simulink model "graph"  (R2015b)
settings: Solver=ode4  StartTime=0.0  StopTime=0.2  FixedStep=0.00002  RelTol=1e-3
settings Model: ExtModeTrigDuration=10000  Creator=husseinz  LastModifiedBy=husseinz
settings SolverCC: PositivePriorityOrder=on
settings RTWCC: SystemTargetFile=quarc_win64.tlc  TemplateMakefile=quarc_default_tmf  Description=QUARC Win64 Target
settings STFCustomTargetCC: TargetPreCompLibLocation=C:\ProgramData\QUARC\lib\2015b\win64\release  GeneratePreprocessorConditionals=Use local settings  CPPClassGenCompliant=off
settings GRTTargetCC: TargetPreCompLibLocation=C:\ProgramData\QUARC\lib\2015b\win64\release  ParMdlRefBuildCompliant=off  CompOptLevelCompliant=off  CombineOutputUpdateFcns=off  MatFileLogging=off  CPPClassGenCompliant=off  GRTInterface=on  UseToolchainInfoCompliant=off  ExtMode=on  ExtModeMexFile=quarc_comm

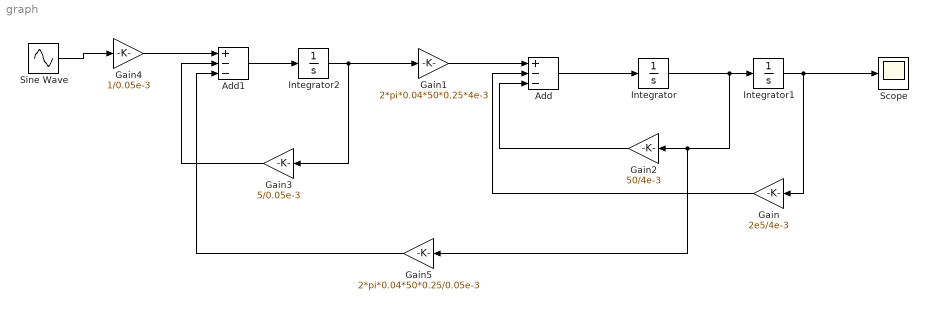
== system graph ==
  Add : Sum  Inputs=+--
  Add1 : Sum  Inputs=+--
  Gain : Gain  Gain=2e5/4e-3
  Gain1 : Gain  Gain=2*pi*0.04*50*0.25*4e-3
  Gain2 : Gain  Gain=50/4e-3
  Gain3 : Gain  Gain=5/0.05e-3
  Gain4 : Gain  Gain=1/0.05e-3
  Gain5 : Gain  Gain=2*pi*0.04*50*0.25/0.05e-3
  Integrator : Integrator
  Integrator1 : Integrator
  Integrator2 : Integrator
  Scope : Scope
  Sine Wave : Sin  Frequency=200  SampleTime=0
  wires:
  Add/1 -> Integrator/1
  Integrator/1 -> Gain5/1, Gain2/1, Integrator1/1
  Integrator1/1 -> Scope/1, Gain/1
  Gain1/1 -> Add/1
  Gain/1 -> Add/2
  Gain2/1 -> Add/3
  Add1/1 -> Integrator2/1
  Integrator2/1 -> Gain1/1, Gain3/1
  Gain3/1 -> Add1/2
  Gain4/1 -> Add1/1
  Sine Wave/1 -> Gain4/1
  Gain5/1 -> Add1/3
